simulink model "trraffic_sys"  (R2020b)
settings: Solver=FixedStepDiscrete  StartTime=0.0  StopTime=150  FixedStep=.1  RelTol=1e-3  EnableMultiTasking=on
undefined symbols (not defined in the file): DiscIntNeverNeededParam
libraries: simulink x1
settings Model: Creator=The MathWorks, Inc.  LastModifiedBy=com
settings DataIOCC: LimitDataPoints=on  SaveFormat=Array  ReturnWorkspaceOutputs=off
settings OptimizationCC: ExpressionDepthLimit=2147483647  InitFltsAndDblsToZero=on  EfficientMapNaN2IntZero=off  LifeSpan=inf
settings DebuggingCC: SaveWithParameterizedLinksMsg=none  UnderspecifiedInitializationDetection=Classic  MergeDetectMultiDrivingBlocksExec=none  SignalResolutionControl=TryResolveAllWithWarning  SolverPrmCheckMsg=warning  MultiTaskDSMMsg=warning  MultiTaskCondExecSysMsg=none  FcnCallInpInsideContextMsg=warning  StateNameClashWarn=warning  SFUnexpectedBacktrackingDiag=warning  SFNoUnconditionalDefaultTransitionDiag=warning  SFExecutionAtInitializationDiag=none  ArithmeticOperatorsInVariantConditions=warning
settings HardwareCC: ProdBitPerPointer=32  ProdBitPerSizeT=32  ProdBitPerPtrDiffT=32  ProdLargestAtomicFloat=None  ProdIntDivRoundTo=Undefined  ProdEndianess=Unspecified  ProdWordSize=32  ProdHWDeviceType=32-bit Generic
settings ModelReferenceCC: PropagateSignalLabelsOutOfModel=off
settings SFSimCC: SimUseLocalCustomCode=off  SimParseCustomCode=off  CustomCodeUndefinedFunction=UseInterfaceOnly
settings RTWCC: RTWUseLocalCustomCode=off
settings CodeAppCC: StateflowObjectComments=on
settings GRTTargetCC: TargetFcnLib=ansi_tfl_tmw.mat  TargetLangStandard=C89/C90 (ANSI)  CombineOutputUpdateFcns=off  GRTInterface=on
settings ConfigComp: CovMetricSettings=dw  CovSaveCumulativeToWorkspaceVar=on  CovSaveSingleToWorkspaceVar=on  CovExternalEMLEnable=off  CovSFcnEnable=off

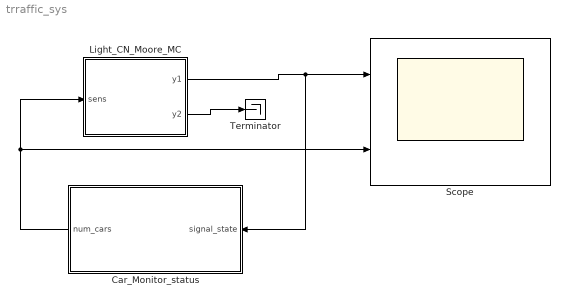
== system trraffic_sys ==
  Car_Monitor_status : Subsystem
  Light_CN_Moore_MC : Stateflow chart  TreatAsAtomicUnit=on
  Scope : Scope  NumInputPorts=2
  Terminator : Terminator
  wires:
  Light_CN_Moore_MC/2(y2) -> Terminator/1
  Car_Monitor_status/1(num_cars) -> Scope/2, Light_CN_Moore_MC/1(sens)
  Light_CN_Moore_MC/1(y1) -> Scope/1, Car_Monitor_status/1(signal_state)

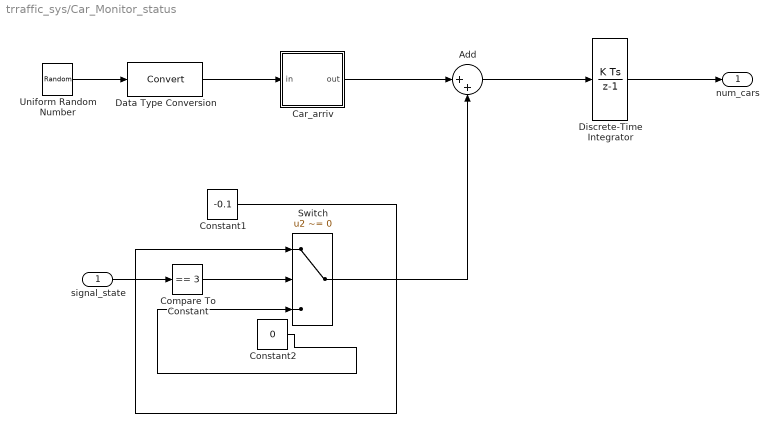
== system trraffic_sys/Car_Monitor_status ==
  signal_state : Inport
  Add : Sum  Inputs=|++
  Car_arriv : Stateflow chart  TreatAsAtomicUnit=on
  Compare To Constant : simulink/Logic and Bit Operations/Compare To Constant  relop===  const=3  OutDataTypeStr=boolean  ZeroCross=off
  Constant1 : Constant  Value=-0.1
  Constant2 : Constant  Value=0
  Data Type Conversion : DataTypeConversion
  Discrete-Time Integrator : DiscreteIntegrator  SampleTime=-1  LimitOutput=on  LowerSaturationLimit=0  ICPrevOutput=DiscIntNeverNeededParam  ICPrevScaledInput=DiscIntNeverNeededParam
  Switch : Switch  Criteria=u2 ~= 0
  Uniform Random Number : UniformRandomNumber  Minimum=0  Maximum=100  Seed=177836  SampleTime=0
  num_cars : Outport  VectorParamsAs1DForOutWhenUnconnected=off
  wires:
  Constant1/1 -> Switch/1
  Constant2/1 -> Switch/3
  signal_state/1 -> Compare To Constant/1
  Compare To Constant/1 -> Switch/2
  Switch/1 -> Add/2
  Add/1 -> Discrete-Time Integrator/1
  Car_arriv/1(out) -> Add/1
  Uniform Random Number/1 -> Data Type Conversion/1
  Discrete-Time Integrator/1 -> num_cars/1
  Data Type Conversion/1 -> Car_arriv/1(in)

== stateflow chart trraffic_sys/Light_CN_Moore_MC ==
  settings: stateMachineType=MOORE_MACHINE  executeAtInitialization=1  initializeOutput=1
  state stopforTraffic
    y1 = red;
    y2 = green;
  state StopToGo
    y1 = red;
    y2 = yellow;
  state stop
    y1 = red;
    y2 = green;
  state GoToStop
    y1 = yellow;
    y2 = red;
  state Go
    y1 = green;
    y2 = red;
  (default) -> stop
  stopforTraffic -> StopToGo : [sens]
  stop -> stopforTraffic : after(20,tick)
  StopToGo -> Go : after(3,tick)
  GoToStop -> stop : after (3,tick)
  Go -> GoToStop : after(10,tick)
  data: sens input double; y1 output double; y2 output double; green constant double =3; red constant double =1; yellow constant double =2

== stateflow chart trraffic_sys/Car_Monitor_status/Car_arriv ==
  (default) -> (junction 2) : {out = in > 98;}
  data: in input int8; out output double
